simulink model "ButtonControlApp"  (R2023a)
settings: Solver=FixedStepDiscrete  StartTime=0.0  StopTime=10.0  FixedStep=0.1  RelTol=1e-3
libraries: androiduilib x6, androidcommunicationlib x1
settings Model: Creator=The MathWorks, Inc.  LastModifiedBy=aqeel
settings SolverCC: AlgebraicLoopSolver=TrustRegion
settings OptimizationCC: EnhancedBackFolding=on  PassReuseOutputArgsThreshold=0  MaxStackSize=64  OptimizeBlockOrder=speed  DifferentSizesBufferReuse=on  OptimizationCustomize=off
settings DebuggingCC: ParameterTunabilityLossMsg=error  UnconnectedInputMsg=warning  UnconnectedOutputMsg=warning  UnconnectedLineMsg=warning  SymbolicDimsDataTypeCodeGenerationDiagnostic=none
settings HardwareCC: ProdBitPerPointer=32  ProdBitPerSizeT=32  ProdBitPerPtrDiffT=32  ProdLargestAtomicInteger=Long  ProdLargestAtomicFloat=Double  ProdWordSize=32  ProdHWDeviceType=ARM Compatible->ARM Cortex  UseEmbeddedCoderFeatures=off  UseSimulinkCoderFeatures=off
settings ModelReferenceCC: EnableRefExpFcnMdlSchedulingChecks=on
settings SFSimCC: MATLABDynamicMemAlloc=off
settings RTWCC: Description=Embedded Coder  SystemTargetFile=ert.tlc  HardwareBoard=Android Device  TLCOptions="-aInlineSetEventsForThisBaseRateFcn=TLC_FALSE -aSuppressMultiTaskScheduler=TLC_FALSE  -aRateBasedStepFcn=0"  TemplateMakefile=ert_default_tmf  GenerateReport=on  RTWVerbose=off  Toolchain=Android SDK/NDK Tools  LaunchReport=on
settings CodeAppCC: ForceParamTrailComments=on  OperatorAnnotations=on
settings ERTTargetCC: ERTCustomFileBanners=off  SupportContinuousTime=on  SupportNonInlinedSFcns=on  RemoveResetFunc=off  ModelStepFunctionPrototypeControlCompliant=off

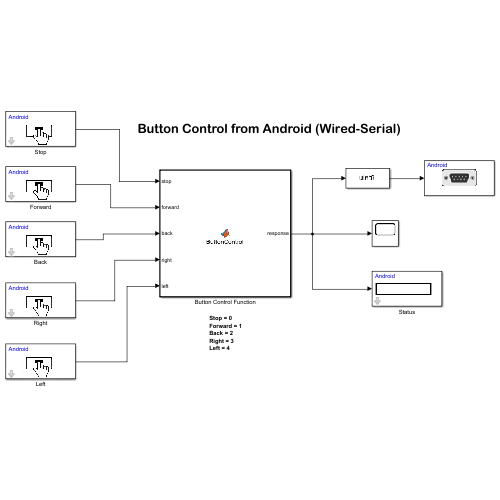
[thumbnail: Simulink's stored preview of the top-level diagram]
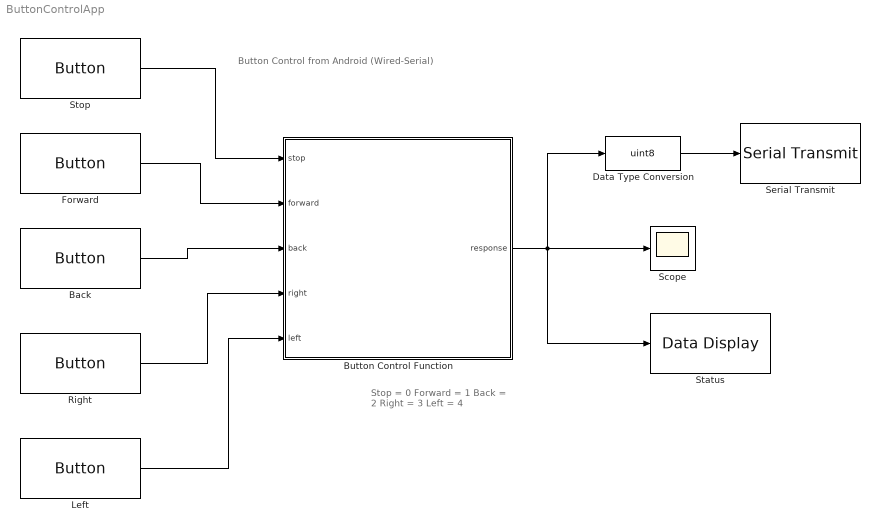
== system ButtonControlApp ==
  note: Button Control from Android (Wired-Serial)
  note: Stop = 0
      | Forward = 1
      | Back = 2
      | Right = 3
      | Left = 4
  Back : androiduilib/Button  ButtonState=Not pressed  ButtonId=ButtonControlApp/Back  State=off  SampleTime=0.1  BlockPlatform=Android
  Button Control Function : MATLAB Function  TreatAsAtomicUnit=on
  Data Type Conversion : DataTypeConversion  OutDataTypeStr=uint8  SaturateOnIntegerOverflow=off  RndMeth=Floor
  Forward : androiduilib/Button  ButtonState=Not pressed  ButtonId=ButtonControlApp/Forward  State=off  SampleTime=0.1  BlockPlatform=Android
  Left : androiduilib/Button  ButtonState=Not pressed  ButtonId=ButtonControlApp/Left  State=off  SampleTime=0.1  BlockPlatform=Android
  Right : androiduilib/Button  ButtonState=Not pressed  ButtonId=ButtonControlApp/Right  State=off  SampleTime=0.1  BlockPlatform=Android
  Scope : Scope
  Serial Transmit : androidcommunicationlib/Serial Transmit
  Status : androiduilib/Data Display  DataDisplayId=ButtonControlApp/Status  Format=Integer  Precision=6  SimulateUsing=Code generation  blockPlatform=Android
  Stop : androiduilib/Button  ButtonState=Not pressed  ButtonId=ButtonControlApp/Stop  State=off  SampleTime=0.1  BlockPlatform=Android
  wires:
  Forward/1 -> Button Control Function/2(forward)
  Stop/1 -> Button Control Function/1(stop)
  Back/1 -> Button Control Function/3(back)
  Right/1 -> Button Control Function/4(right)
  Left/1 -> Button Control Function/5(left)
  Button Control Function/1(response) -> Data Type Conversion/1, Status/1, Scope/1
  Data Type Conversion/1 -> Serial Transmit/1

== matlab function ButtonControlApp/Button Control Function ==
  data: stop input; response output; forward input; back input; right input; left input
%Function to control Arduino robot using the android device
%Robot Controls:
%response = 0 --> Stop
%response = 1 --> Forward
%response = 2 --> Reverse
%response = 3 --> Right
%response = 4 --> Left

function response = ButtonControl(stop,forward,back,right,left)
Buttons=[stop,forward,back,right,left];
if sum(Buttons)==1
    if stop == 1
        response = 0;
    elseif forward==1
        response =1;
    elseif back ==1
        response=2;
    elseif right ==1
        response=3;
    elseif left==1
        response=4;
    else
        response=0;
    end
else
    response=0;
end
